simulink model "HighPassFilter_Bilinear"  (R2020b)
settings: Solver=VariableStepAuto  StartTime=0.0  StopTime=10.0  RelTol=1e-3
settings Model: Creator=Admin  LastModifiedBy=Admin

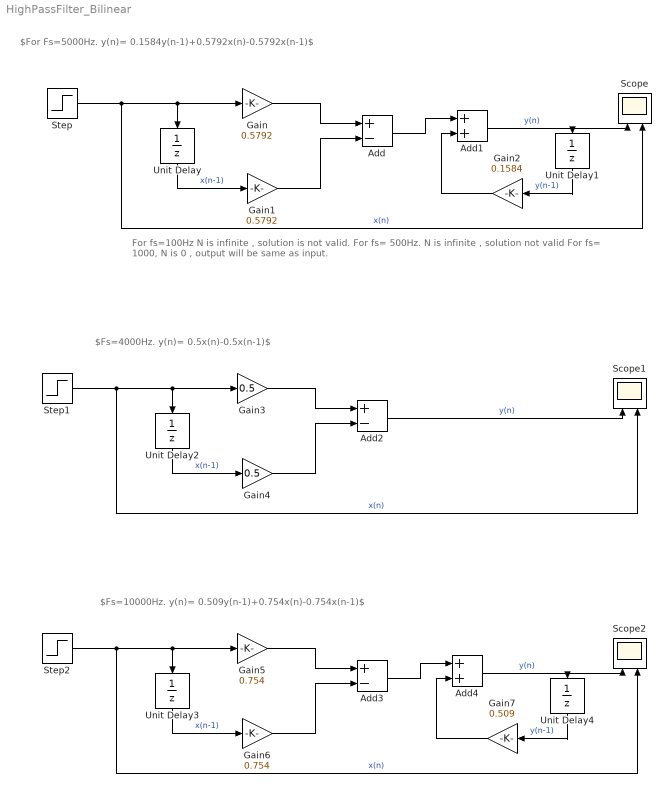
== system HighPassFilter_Bilinear ==
  note: $Fs=10000Hz. y(n)= 0.509y(n-1)+0.754x(n)-0.754x(n-1)$
  note: $Fs=4000Hz. y(n)= 0.5x(n)-0.5x(n-1)$
  note: $For Fs=5000Hz. y(n)= 0.1584y(n-1)+0.5792x(n)-0.5792x(n-1)$
  note: For fs=100Hz N is infinite , solution is not valid.
      | For fs= 500Hz. N is infinite , solution not valid
      | For fs= 1000, N is 0 , output will be same as input.
  Add : Sum  Inputs=+-
  Add1 : Sum
  Add2 : Sum  Inputs=+-
  Add3 : Sum  Inputs=+-
  Add4 : Sum
  Gain : Gain  Gain=0.5792
  Gain1 : Gain  Gain=0.5792
  Gain2 : Gain  Gain=0.1584
  Gain3 : Gain  Gain=0.5
  Gain4 : Gain  Gain=0.5
  Gain5 : Gain  Gain=0.754
  Gain6 : Gain  Gain=0.754
  Gain7 : Gain  Gain=0.509
  Scope : Scope  NumInputPorts=2
  Scope1 : Scope  NumInputPorts=2
  Scope2 : Scope  NumInputPorts=2
  Step : Step  SampleTime=0
  Step1 : Step  SampleTime=0
  Step2 : Step  SampleTime=0
  Unit Delay{,1..4} (5 alike) : UnitDelay  SampleTime=-1  HasFrameUpgradeWarning=on
  wires:
  Unit Delay2/1 -> Gain4/1  "x(n-1)"
  Step1/1 -> Gain3/1, Unit Delay2/1, Scope1/2  "x(n)"
  Gain4/1 -> Add2/2
  Add/1 -> Add1/1
  Unit Delay4/1 -> Gain7/1  "y(n-1)"
  Add1/1 -> Scope/1, Unit Delay1/1  "y(n)"
  Unit Delay1/1 -> Gain2/1  "y(n-1)"
  Gain6/1 -> Add3/2
  Unit Delay3/1 -> Gain6/1  "x(n-1)"
  Gain3/1 -> Add2/1
  Add4/1 -> Scope2/1, Unit Delay4/1  "y(n)"
  Gain7/1 -> Add4/2
  Gain5/1 -> Add3/1
  Add2/1 -> Scope1/1  "y(n)"
  Add3/1 -> Add4/1
  Gain/1 -> Add/1
  Step/1 -> Gain/1, Unit Delay/1, Scope/2  "x(n)"
  Unit Delay/1 -> Gain1/1  "x(n-1)"
  Gain2/1 -> Add1/2
  Gain1/1 -> Add/2
  Step2/1 -> Gain5/1, Unit Delay3/1, Scope2/2  "x(n)"
